simulink model "second_order"  (R2022b)
settings: Solver=VariableStepAuto  StartTime=0.0  StopTime=1  RelTol=1e-3
model workspace (MAT data in the model file):
  Sig = Simulink.Signal
  Sig.DataType = 'auto'
  Sig.Dimensions = -1
  Sig.DimensionsMode = 'auto'
  Sig.Complexity = 'auto'
  Sig.SampleTime = -1
  Sig.SamplingMode = 'auto'
  a1 = -0.1406
  a2 = -0.6892
  b1 = 0.1406
  b2 = 0.6892
  b3 = 0
  c1 = 5.513
  c2 = 0.0569
  g1 = -0.00088168
libraries: simulink_extras x1, eeGeneralControl x1
settings Model: Creator=ge95yur  LastModifiedBy=94749
settings DebuggingCC: UnconnectedInputMsg=warning  UnconnectedOutputMsg=warning  UnconnectedLineMsg=warning
settings ModelReferenceCC: EnableRefExpFcnMdlSchedulingChecks=on
settings RTWCC: DLArmComputeVersion=19.05

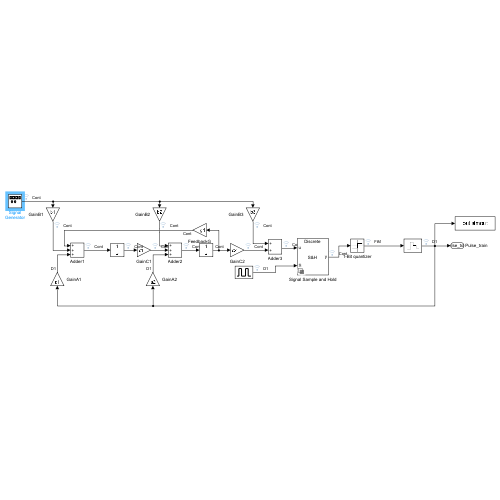
[thumbnail: Simulink's stored preview of the top-level diagram]
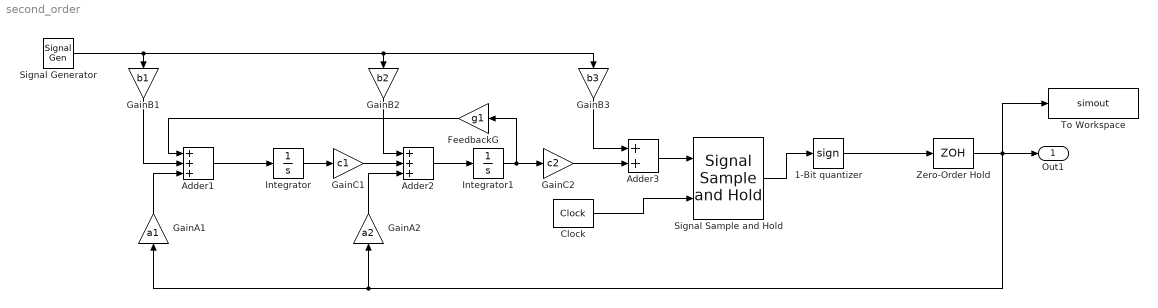
== system second_order ==
  1-Bit quantizer : Signum
  Adder1 : Sum  Inputs=+++
  Adder2 : Sum  Inputs=+++
  Adder3 : Sum
  Clock : simulink_extras/Flip Flops/Clock  period=1/(256*2*1e4)
  FeedbackG : Gain  Gain=g1
  GainA1 : Gain  Gain=a1
  GainA2 : Gain  Gain=a2
  GainB1 : Gain  Gain=b1
  GainB2 : Gain  Gain=b2
  GainB3 : Gain  Gain=b3
  GainC1 : Gain  Gain=c1
  GainC2 : Gain  Gain=c2
  Integrator : Integrator
  Integrator1 : Integrator
  Signal Generator : SignalGenerator  Amplitude=0.5  Frequency=1e2
  Signal Sample and Hold : eeGeneralControl/Signal Sample and Hold  LabelModeActiveChoice=Discrete  x0=0  Ts=-1
  To Workspace : ToWorkspace  VariableName=simout  SaveFormat=Timeseries  SampleTime=-1
  Zero-Order Hold : ZeroOrderHold  SampleTime=-1
  Out1 : Outport  SignalName=Pulse_train
  wires:
  Integrator/1 -> GainC1/1
  GainC1/1 -> Adder2/2
  Adder2/1 -> Integrator1/1
  Integrator1/1 -> GainC2/1, FeedbackG/1
  GainC2/1 -> Adder3/2
  GainB3/1 -> Adder3/1
  GainB2/1 -> Adder2/1
  Adder1/1 -> Integrator/1
  GainB1/1 -> Adder1/2
  FeedbackG/1 -> Adder1/1
  GainA1/1 -> Adder1/3
  GainA2/1 -> Adder2/3
  Signal Generator/1 -> GainB2/1, GainB3/1, GainB1/1
  Signal Sample and Hold/1 -> 1-Bit quantizer/1
  Zero-Order Hold/1 -> To Workspace/1, Out1/1, GainA2/1, GainA1/1
  Adder3/1 -> Signal Sample and Hold/1
  Clock/1 -> Signal Sample and Hold/2
  1-Bit quantizer/1 -> Zero-Order Hold/1
